simulink model "six_model"  (R2021b)
settings: Solver=VariableStepAuto  StartTime=0.0  StopTime=10.0  RelTol=1e-3
values from neighbouring files (symbols this model uses):
  A = [ 0 1 0; 12.077 -0.0014 0.1407; 0 0 -0.2606]    [Project_part_2_code.m]
  B = [0; -0.0281; 0.0519]    [Project_part_2_code.m]
  k = acker(A,B,p)    [Project_part_2_code.m]
undefined symbols (not defined in the file or in its folder): E
settings Model: Creator=chand  LastModifiedBy=chand

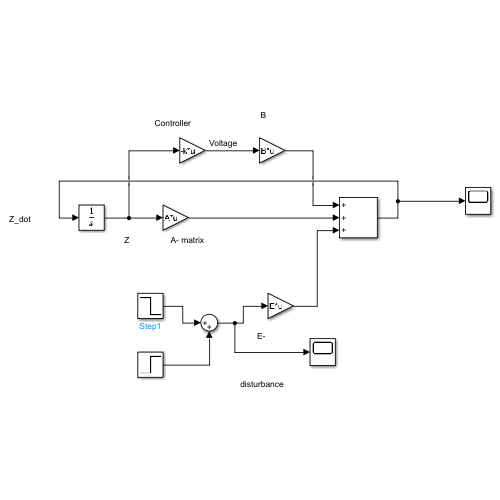
[thumbnail: Simulink's stored preview of the top-level diagram]
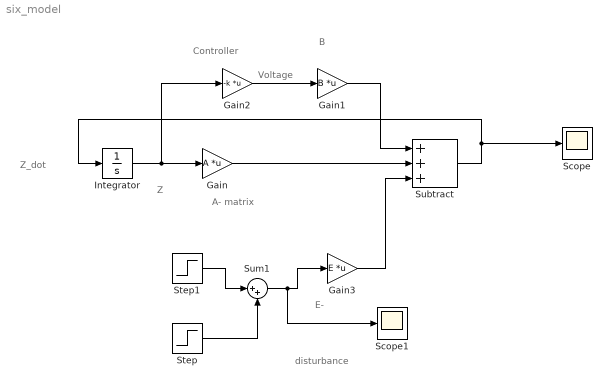
== system six_model ==
  note: Controller
  note: Z
  note: B
  note: disturbance
  note: E-
  note: Voltage
  note: A- matrix
  note: Z_dot
  Gain : Gain  Gain=A  Multiplication=Matrix(K*u)
  Gain1 : Gain  Gain=B  Multiplication=Matrix(K*u)
  Gain2 : Gain  Gain=-k  Multiplication=Matrix(K*u)
  Gain3 : Gain  Gain=E  Multiplication=Matrix(K*u)
  Integrator : Integrator
  Scope : Scope
  Scope1 : Scope
  Step : Step  Time=0  SampleTime=0
  Step1 : Step  After=-1  SampleTime=0
  Subtract : Sum  Inputs=+++
  Sum1 : Sum  Inputs=|++
  wires:
  Subtract/1 -> Integrator/1, Scope/1
  Gain2/1 -> Gain1/1
  Integrator/1 -> Gain2/1, Gain/1
  Gain/1 -> Subtract/2
  Gain3/1 -> Subtract/3
  Gain1/1 -> Subtract/1
  Step1/1 -> Sum1/1
  Step/1 -> Sum1/2
  Sum1/1 -> Scope1/1, Gain3/1
